simulink model "UPQC_model"  (R2020b)
settings: Solver=FixedStepAuto  StartTime=0.0  StopTime=Tsim  FixedStep=Tsample  MaxStep=Tsample  RelTol=1e-3
values from neighbouring files (symbols this model uses):
  C_parallel_Series = zeros(1,4)    [Netzmodell_Ini_DL.m]    (also in workspace_Ini.mat = [1e-05 1e-05 1e-05 0])
  C_parallel_Shunt = zeros(1,4)    [Netzmodell_Ini_DL.m]    (also in workspace_Ini.mat = [1e-05 1e-05 1e-05 0])
  CC_Ki = 5    [Netzmodell_Ini_DL.m]    (also in workspace_Ini.mat)
  CC_Ki_geg = 5    [Netzmodell_Ini_DL.m]    (also in workspace_Ini.mat)
  CC_Kp = 10    [Netzmodell_Ini_DL.m]    (also in workspace_Ini.mat)
  CC_Kp_geg = 10    [Netzmodell_Ini_DL.m]    (also in workspace_Ini.mat)
  CC_OS =     [workspace_Ini.mat]
  Czk = Szenario.Czk*u    [Netzmodell_Ini_DL.m]    (also in workspace_Ini.mat = 0.003)
  fak_RVC = Szenario.fak_RVC    [Netzmodell_Ini_DL.m]    (also in workspace_Ini.mat = [1 1 1])
  fak_Uns = [1; 1; 1]    [Netzmodell_Ini_DL.m]    (also in workspace_Ini.mat = [1 1 1])
  Flicker_Schaltzeitpunkte_L1 = Schaltzeitpunkte(1,:)    [Netzmodell_Ini_DL.m]    (also in workspace_Ini.mat = 10.5)
  Flicker_Schaltzeitpunkte_L2 = Schaltzeitpunkte(2,:)    [Netzmodell_Ini_DL.m]    (also in workspace_Ini.mat = 10.5)
  Flicker_Schaltzeitpunkte_L3 = Schaltzeitpunkte(3,:)    [Netzmodell_Ini_DL.m]    (also in workspace_Ini.mat = 10.5)
  fs = [f_nom; f_nom; f_nom]    [Netzmodell_Ini_DL.m]    (also in workspace_Ini.mat = [50 50 50])
  fsw = Szenario.fsw*k    [Netzmodell_Ini_DL.m]    (also in workspace_Ini.mat = 20000)
  I_Basis_Ober_L1 = I_Basis_Ober(1)    [Netzmodell_Ini_DL.m]    (also in workspace_Ini.mat = 0)
  I_Basis_Ober_L2 = I_Basis_Ober(2)    [Netzmodell_Ini_DL.m]    (also in workspace_Ini.mat = 0)
  I_Basis_Ober_L3 = I_Basis_Ober(3)    [Netzmodell_Ini_DL.m]    (also in workspace_Ini.mat = 0)
  I_relativ_Ober_L1 = Szenario.I_relativ_Ober_L1    [Netzmodell_Ini_DL.m]    (also in workspace_Ini.mat = [0 100 0 100 100 0 100 100 0 0 0 0 ... (50 elements, 1x50)])
  I_relativ_Ober_L2 = Szenario.I_relativ_Ober_L2    [Netzmodell_Ini_DL.m]    (also in workspace_Ini.mat = [0 100 0 100 100 0 100 100 0 0 0 0 ... (50 elements, 1x50)])
  I_relativ_Ober_L3 = Szenario.I_relativ_Ober_L3    [Netzmodell_Ini_DL.m]    (also in workspace_Ini.mat = [0 100 0 100 100 0 100 100 0 0 0 0 ... (50 elements, 1x50)])
  L_Ausgang_Series = zeros(1,4)    [Netzmodell_Ini_DL.m]    (also in workspace_Ini.mat = [0.00093 0.00093 0.00093 0.00093])
  L_Ausgang_Shunt = zeros(1,4)    [Netzmodell_Ini_DL.m]    (also in workspace_Ini.mat = [0.00093 0.00093 0.00093 0.00093])
  L_Eingang_Series = zeros(1,4)    [Netzmodell_Ini_DL.m]    (also in workspace_Ini.mat = [0.00085 0.00085 0.00085 0.00085])
  L_Eingang_Shunt = zeros(1,4)    [Netzmodell_Ini_DL.m]    (also in workspace_Ini.mat = [0.00085 0.00085 0.00085 0.00085])
  Ls_in = 52.2*u/10    (= 5.22e-06)    [Netzmodell_Ini_DL.m]    (also in workspace_Ini.mat)
  Ltrans = Szenario.Ltrans*m    [Netzmodell_Ini_DL.m]    (also in workspace_Ini.mat = 0.000256)
  OS_off = 6    [Netzmodell_Ini_DL.m]    (also in workspace_Ini.mat)
  OS_on = 1    [Netzmodell_Ini_DL.m]    (also in workspace_Ini.mat)
  Phi_Ober_L1 = Phi_Ober(1)    [Netzmodell_Ini_DL.m]    (also in workspace_Ini.mat = 0)
  Phi_Ober_L2 = Phi_Ober(2)    [Netzmodell_Ini_DL.m]    (also in workspace_Ini.mat = -120)
  Phi_Ober_L3 = Phi_Ober(3)    [Netzmodell_Ini_DL.m]    (also in workspace_Ini.mat = 120)
  Phis = [0; -120; 120]    [Netzmodell_Ini_DL.m]    (also in workspace_Ini.mat = [0 -120 120])
  Pl_Flicker = Pl_Flicker*k    [Netzmodell_Ini_DL.m]    (also in workspace_Ini.mat = [5000 5000 5000])
  Pl_Grund = Szenario.Pl_Grund *k    [Netzmodell_Ini_DL.m]    (also in workspace_Ini.mat = [5 5 5])
  Pl_RVC = Pl_RVC*k    [Netzmodell_Ini_DL.m]    (also in workspace_Ini.mat = [10000 10000 10000])
  Pl_Uns = Pl_Uns*k    [Netzmodell_Ini_DL.m]    (also in workspace_Ini.mat = [25000 10 10])
  Ql_ind_Flicker = Ql_ind_Flicker*k    [Netzmodell_Ini_DL.m]    (also in workspace_Ini.mat = [0 0 0])
  Ql_ind_Grund = Szenario.Ql_ind_Grund*k    [Netzmodell_Ini_DL.m]    (also in workspace_Ini.mat = [0 0 0])
  Ql_ind_RVC = Szenario.Ql_ind_RVC*k    [Netzmodell_Ini_DL.m]    (also in workspace_Ini.mat = [0 0 0])
  Ql_ind_Uns = Ql_ind_Uns*k    [Netzmodell_Ini_DL.m]    (also in workspace_Ini.mat = [0 0 0])
  Ql_kap_Flicker = Ql_kap_Flicker*k    [Netzmodell_Ini_DL.m]    (also in workspace_Ini.mat = [0 0 0])
  Ql_kap_Grund = Szenario.Ql_kap_Grund*k    [Netzmodell_Ini_DL.m]    (also in workspace_Ini.mat = [0 0 0])
  Ql_kap_RVC = Szenario.Ql_kap_RVC*k    [Netzmodell_Ini_DL.m]    (also in workspace_Ini.mat = [0 0 0])
  Ql_kap_Uns = Ql_kap_Uns*k    [Netzmodell_Ini_DL.m]    (also in workspace_Ini.mat = [0 0 0])
  R_Ausgang_Series = zeros(1,4)    [Netzmodell_Ini_DL.m]    (also in workspace_Ini.mat = [0.1 0.1 0.1 0.1])
  R_Ausgang_Shunt = zeros(1,4)    [Netzmodell_Ini_DL.m]    (also in workspace_Ini.mat = [0.1 0.1 0.1 0.1])
  R_Eingang_Series = zeros(1,4)    [Netzmodell_Ini_DL.m]    (also in workspace_Ini.mat = [0.1 0.1 0.1 0.1])
  R_Eingang_Shunt = zeros(1,4)    [Netzmodell_Ini_DL.m]    (also in workspace_Ini.mat = [0.1 0.1 0.1 0.1])
  R_parallel_Series = zeros(1,4)    [Netzmodell_Ini_DL.m]    (also in workspace_Ini.mat = [13 13 13 0])
  R_parallel_Shunt = zeros(1,4)    [Netzmodell_Ini_DL.m]    (also in workspace_Ini.mat = [13 13 13 0])
  R_ZK_Belastung = 20    [Netzmodell_Ini_DL.m]    (also in workspace_Ini.mat)
  Rs_in = 5.2*m/10    (= 0.00052)    [Netzmodell_Ini_DL.m]    (also in workspace_Ini.mat)
  Rtrans = Szenario.Rtrans    [Netzmodell_Ini_DL.m]    (also in workspace_Ini.mat = 0.206)
  RVC_L1_on_off_Zeitpunkte = Szenario.RVC_L1_on_off_Zeitpunkte    [Netzmodell_Ini_DL.m]    (also in workspace_Ini.mat = [10.5 40 10 11 12 13 14 15])
  RVC_L2_on_off_Zeitpunkte = Szenario.RVC_L2_on_off_Zeitpunkte    [Netzmodell_Ini_DL.m]    (also in workspace_Ini.mat = [10.5 40 10 11 12 13 14 15])
  RVC_L3_on_off_Zeitpunkte = Szenario.RVC_L3_on_off_Zeitpunkte    [Netzmodell_Ini_DL.m]    (also in workspace_Ini.mat = [10.5 40 10 11 12 13 14 15])
  RVC_off = 20.5    [Netzmodell_Ini_DL.m]    (also in workspace_Ini.mat)
  RVC_on = 20    [Netzmodell_Ini_DL.m]    (also in workspace_Ini.mat)
  RVC_val = [0.8,0.8,0.8]    [Netzmodell_Ini_DL.m]    (also in workspace_Ini.mat = [0.8 0.8 0.8])
  strans = Szenario.strans    [Netzmodell_Ini_DL.m]    (also in workspace_Ini.mat = 0.25)
  t_breaker_series = tacts    [Netzmodell_Ini_DL.m]    (also in workspace_Ini.mat = 0.5)
  tact = Szenario.tact    [Netzmodell_Ini_DL.m]    (also in workspace_Ini.mat = 0.5)
  tact_OS_Regler = Szenario.tact_OS_Regler    [Netzmodell_Ini_DL.m]    (also in workspace_Ini.mat = 0.5)
  tact_QU = 10    [Netzmodell_Ini_DL.m]    (also in workspace_Ini.mat)
  tacts = Szenario.tacts    [Netzmodell_Ini_DL.m]    (also in workspace_Ini.mat = 0.5)
  Tsample = Szenario.Tsample    [Netzmodell_Ini_DL.m]    (also in workspace_Ini.mat = 5e-06)
  Uns_L1_on_off_Zeitpunkte = Szenario.Uns_L1_on_off_Zeitpunkte    [Netzmodell_Ini_DL.m]    (also in workspace_Ini.mat = [1 6 10 11 12 13 14 15])
  Uns_L2_on_off_Zeitpunkte = Szenario.Uns_L2_on_off_Zeitpunkte    [Netzmodell_Ini_DL.m]    (also in workspace_Ini.mat = [10 30 10 11 12 13 14 15])
  Uns_L3_on_off_Zeitpunkte = Szenario.Uns_L3_on_off_Zeitpunkte    [Netzmodell_Ini_DL.m]    (also in workspace_Ini.mat = [10 30 10 11 12 13 14 15])
  Us = [Us_Amp; Us_Amp; Us_Amp]    [Netzmodell_Ini_DL.m]    (also in workspace_Ini.mat = [326.598632371 326.598632371 326.598632371])
  Us_Amp = sqrt(2)*400/sqrt(3)    [Netzmodell_Ini_DL.m]    (also in workspace_Ini.mat = 326.598632371)
  VC_Ki_gegen = 30    [Netzmodell_Ini_DL.m]    (also in workspace_Ini.mat)
  VC_Ki_gegen_shunt = 15    [Netzmodell_Ini_DL.m]    (also in workspace_Ini.mat)
  VC_Ki_mit = 5    [Netzmodell_Ini_DL.m]    (also in workspace_Ini.mat)
  VC_Kp_gegen = 5    [workspace_Ini.mat]
  VC_Kp_gegen_shunt = 2    [Netzmodell_Ini_DL.m]    (also in workspace_Ini.mat)
  VC_Kp_mit = 10    [Netzmodell_Ini_DL.m]    (also in workspace_Ini.mat)
  VC_ZK_Ki = 5    [Netzmodell_Ini_DL.m]    (also in workspace_Ini.mat)
  VC_ZK_Kp = 0.5    [Netzmodell_Ini_DL.m]    (also in workspace_Ini.mat)
  Vielfache_Ober_L1 = Szenario.Vielfache_Ober_L1    [Netzmodell_Ini_DL.m]    (also in workspace_Ini.mat = [1 2 3 4 5 6 7 8 9 10 11 12 ... (50 elements, 1x50)])
  Vielfache_Ober_L2 = Szenario.Vielfache_Ober_L2    [Netzmodell_Ini_DL.m]    (also in workspace_Ini.mat = [1 2 3 4 5 6 7 8 9 10 11 12 ... (50 elements, 1x50)])
  Vielfache_Ober_L3 = Szenario.Vielfache_Ober_L3    [Netzmodell_Ini_DL.m]    (also in workspace_Ini.mat = [1 2 3 4 5 6 7 8 9 10 11 12 ... (50 elements, 1x50)])
  ZK_Belastung_off = 100    [Netzmodell_Ini_DL.m]    (also in workspace_Ini.mat)
  ZK_Belastung_on = 100    [Netzmodell_Ini_DL.m]    (also in workspace_Ini.mat)
  Zwischenkreisspannung = 700    [Netzmodell_Ini_DL.m]    (also in workspace_Ini.mat)
undefined symbols (not defined in the file or in its folder): LAusgang, RReiheL3
libraries: powerlib x221, powerlib_meascontrol x80, pid_lib x23, eeTransforms x4, eePwmGeneratorTwoLevel x2, dspstat3 x1
(part 3 of 16)

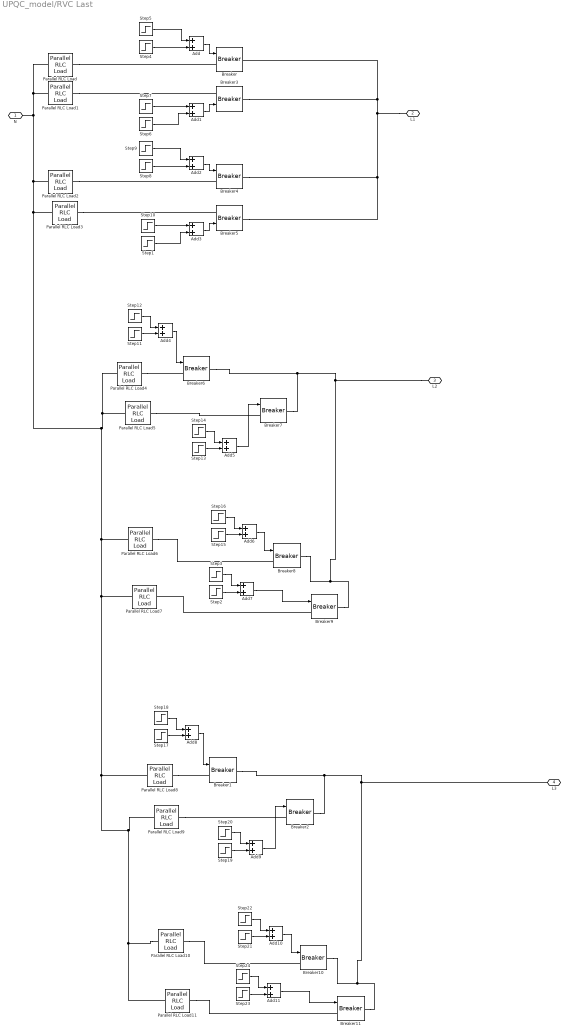
== system UPQC_model/RVC Last ==
  Add{,1..11} (12 alike) : Sum
  Breaker{,1..11} (12 alike) : powerlib/Elements/Breaker  InitialState=0  SwitchingTimes="[1/60  5/60]"  External=on  BreakerResistance=0.01  SnubberResistance=1e6  SnubberCapacitance=inf  Measurements=None  MoreParameters=on  NoBreakLoop=off
  Parallel RLC Load : powerlib/Elements/Parallel RLC Load  LConnTagsString=a  RConnTagsString=__new0  NominalVoltage=230.9  NominalFrequency=50  ActivePower=wirk_L1  InductivePower=blind_ind_L1  CapacitivePower=blind_kap_L1  Setx0=off  InitialVoltage=0  SetiL0=off  InitialCurrent=0  Measurements=None  LoadType=constant Z
      settings: AttributesFormatString=\n  SourceProductBaseCode=PS
  Parallel RLC Load1 : powerlib/Elements/Parallel RLC Load  LConnTagsString=a  RConnTagsString=__new0  NominalVoltage=230.9  NominalFrequency=50  ActivePower=wirk_L1*faktor_L1  InductivePower=blind_ind_L1*faktor_L1  CapacitivePower=blind_kap_L1*faktor_L1  Setx0=off  InitialVoltage=0  SetiL0=off  InitialCurrent=0  Measurements=None  LoadType=constant Z
      settings: AttributesFormatString=\n  SourceProductBaseCode=PS
  Parallel RLC Load10 : powerlib/Elements/Parallel RLC Load  LConnTagsString=a  RConnTagsString=__new0  NominalVoltage=230.9  NominalFrequency=50  ActivePower=wirk_L3*faktor_L3*faktor_L3  InductivePower=blind_ind_L3*faktor_L3*faktor_L3  CapacitivePower=blind_kap_L3*faktor_L3*faktor_L3  Setx0=off  InitialVoltage=0  SetiL0=off  InitialCurrent=0  Measurements=None  LoadType=constant Z
      settings: AttributesFormatString=\n  SourceProductBaseCode=PS
  Parallel RLC Load11 : powerlib/Elements/Parallel RLC Load  LConnTagsString=a  RConnTagsString=__new0  NominalVoltage=230.9  NominalFrequency=50  ActivePower=wirk_L3*faktor_L3*faktor_L3*faktor_L3  InductivePower=blind_ind_L3*faktor_L3*faktor_L3*faktor_L3  CapacitivePower=blind_kap_L3*faktor_L3*faktor_L3*faktor_L3  Setx0=off  InitialVoltage=0  SetiL0=off  InitialCurrent=0  Measurements=None  LoadType=constant Z
      settings: AttributesFormatString=\n  SourceProductBaseCode=PS
  Parallel RLC Load2 : powerlib/Elements/Parallel RLC Load  LConnTagsString=a  RConnTagsString=__new0  NominalVoltage=230.9  NominalFrequency=50  ActivePower=wirk_L1*faktor_L1*faktor_L1  InductivePower=blind_ind_L1*faktor_L1*faktor_L1  CapacitivePower=blind_kap_L1*faktor_L1*faktor_L1  Setx0=off  InitialVoltage=0  SetiL0=off  InitialCurrent=0  Measurements=None  LoadType=constant Z
      settings: AttributesFormatString=\n  SourceProductBaseCode=PS
  Parallel RLC Load3 : powerlib/Elements/Parallel RLC Load  LConnTagsString=a  RConnTagsString=__new0  NominalVoltage=230.9  NominalFrequency=50  ActivePower=wirk_L1*faktor_L1*faktor_L1*faktor_L1  InductivePower=blind_ind_L1*faktor_L1*faktor_L1*faktor_L1  CapacitivePower=blind_kap_L1*faktor_L1*faktor_L1*faktor_L1  Setx0=off  InitialVoltage=0  SetiL0=off  InitialCurrent=0  Measurements=None  LoadType=constant Z
      settings: AttributesFormatString=\n  SourceProductBaseCode=PS
  Parallel RLC Load4 : powerlib/Elements/Parallel RLC Load  LConnTagsString=a  RConnTagsString=__new0  NominalVoltage=230.9  NominalFrequency=50  ActivePower=wirk_L2  InductivePower=blind_ind_L2  CapacitivePower=blind_kap_L2  Setx0=off  InitialVoltage=0  SetiL0=off  InitialCurrent=0  Measurements=None  LoadType=constant Z
      settings: AttributesFormatString=\n  SourceProductBaseCode=PS
  Parallel RLC Load5 : powerlib/Elements/Parallel RLC Load  LConnTagsString=a  RConnTagsString=__new0  NominalVoltage=230.9  NominalFrequency=50  ActivePower=wirk_L2*faktor_L2  InductivePower=blind_ind_L2*faktor_L2  CapacitivePower=blind_kap_L2*faktor_L2  Setx0=off  InitialVoltage=0  SetiL0=off  InitialCurrent=0  Measurements=None  LoadType=constant Z
      settings: AttributesFormatString=\n  SourceProductBaseCode=PS
  Parallel RLC Load6 : powerlib/Elements/Parallel RLC Load  LConnTagsString=a  RConnTagsString=__new0  NominalVoltage=230.9  NominalFrequency=50  ActivePower=wirk_L2*faktor_L2*faktor_L2  InductivePower=blind_ind_L2*faktor_L2*faktor_L2  CapacitivePower=blind_kap_L2*faktor_L2*faktor_L2  Setx0=off  InitialVoltage=0  SetiL0=off  InitialCurrent=0  Measurements=None  LoadType=constant Z
      settings: AttributesFormatString=\n  SourceProductBaseCode=PS
  Parallel RLC Load7 : powerlib/Elements/Parallel RLC Load  LConnTagsString=a  RConnTagsString=__new0  NominalVoltage=230.9  NominalFrequency=50  ActivePower=wirk_L2*faktor_L2*faktor_L2*faktor_L2  InductivePower=blind_ind_L2*faktor_L2*faktor_L2*faktor_L2  CapacitivePower=blind_kap_L2*faktor_L2*faktor_L2*faktor_L2  Setx0=off  InitialVoltage=0  SetiL0=off  InitialCurrent=0  Measurements=None  LoadType=constant Z
      settings: AttributesFormatString=\n  SourceProductBaseCode=PS
  Parallel RLC Load8 : powerlib/Elements/Parallel RLC Load  LConnTagsString=a  RConnTagsString=__new0  NominalVoltage=230.9  NominalFrequency=50  ActivePower=wirk_L3  InductivePower=blind_ind_L3  CapacitivePower=blind_kap_L3  Setx0=off  InitialVoltage=0  SetiL0=off  InitialCurrent=0  Measurements=None  LoadType=constant Z
      settings: AttributesFormatString=\n  SourceProductBaseCode=PS
  Parallel RLC Load9 : powerlib/Elements/Parallel RLC Load  LConnTagsString=a  RConnTagsString=__new0  NominalVoltage=230.9  NominalFrequency=50  ActivePower=wirk_L3*faktor_L3  InductivePower=blind_ind_L3*faktor_L3  CapacitivePower=blind_kap_L3*faktor_L3  Setx0=off  InitialVoltage=0  SetiL0=off  InitialCurrent=0  Measurements=None  LoadType=constant Z
      settings: AttributesFormatString=\n  SourceProductBaseCode=PS
  Step1 : Step  Time=t4_L1  SampleTime=0
  Step10 : Step  Time=t4_L1+(t4_L1_off-t4_L1)  After=-1  SampleTime=0
  Step11 : Step  Time=t1_L2  SampleTime=0
  Step12 : Step  Time=t1_L2+(t1_L2_off-t1_L2)  After=-1  SampleTime=0
  Step13 : Step  Time=t2_L2  SampleTime=0
  Step14 : Step  Time=t2_L2+(t2_L2_off-t2_L2)  After=-1  SampleTime=0
  Step15 : Step  Time=t3_L2  SampleTime=0
  Step16 : Step  Time=t3_L2+(t3_L2_off-t3_L2)  After=-1  SampleTime=0
  Step17 : Step  Time=t1_L3  SampleTime=0
  Step18 : Step  Time=t1_L3+(t1_L3_off-t1_L3)  After=-1  SampleTime=0
  Step19 : Step  Time=t2_L3  SampleTime=0
  Step2 : Step  Time=t4_L2  SampleTime=0
  Step20 : Step  Time=t2_L3+(t2_L3_off-t2_L3)  After=-1  SampleTime=0
  Step21 : Step  Time=t3_L3  SampleTime=0
  Step22 : Step  Time=t3_L3+(t3_L3_off-t3_L3)  After=-1  SampleTime=0
  Step23 : Step  Time=t4_L3  SampleTime=0
  Step24 : Step  Time=t4_L3+(t4_L3_off-t4_L3)  After=-1  SampleTime=0
  Step3 : Step  Time=t4_L2+(t4_L2_off-t4_L2)  After=-1  SampleTime=0
  Step4 : Step  Time=t1_L1  SampleTime=0
  Step5 : Step  Time=t1_L1+(t1_L1_off-t1_L1)  After=-1  SampleTime=0
  Step6 : Step  Time=t2_L1  SampleTime=0
  Step7 : Step  Time=t2_L1+(t2_L1_off-t2_L1)  After=-1  SampleTime=0
  Step8 : Step  Time=t3_L1  SampleTime=0
  Step9 : Step  Time=t3_L1+(t3_L1_off-t3_L1)  After=-1  SampleTime=0
  N : PMIOPort  Side=Left
  L1 : PMIOPort  Port=2  Side=Right
  L2 : PMIOPort  Port=3  Side=Right
  L3 : PMIOPort  Port=4  Side=Right
  wires:
  Step19/1 -> Add9/2
  Step18/1 -> Add8/1
  Step22/1 -> Add10/1
  Step24/1 -> Add11/1
  Step21/1 -> Add10/2
  Add8/1 -> Breaker1/1
  Add11/1 -> Breaker11/1
  Step23/1 -> Add11/2
  Add9/1 -> Breaker2/1
  Step20/1 -> Add9/1
  Step17/1 -> Add8/2
  Add10/1 -> Breaker10/1
  Step11/1 -> Add4/2
  Step14/1 -> Add5/1
  Step13/1 -> Add5/2
  Add6/1 -> Breaker8/1
  Step15/1 -> Add6/2
  Step12/1 -> Add4/1
  Add4/1 -> Breaker6/1
  Add7/1 -> Breaker9/1
  Step16/1 -> Add6/1
  Add5/1 -> Breaker7/1
  Step2/1 -> Add7/2
  Step3/1 -> Add7/1
  Add3/1 -> Breaker5/1
  Step1/1 -> Add3/2
  Step10/1 -> Add3/1
  Add2/1 -> Breaker4/1
  Step8/1 -> Add2/2
  Step9/1 -> Add2/1
  Step7/1 -> Add1/1
  Step6/1 -> Add1/2
  Add1/1 -> Breaker3/1
  Add/1 -> Breaker/1
  Step4/1 -> Add/2
  Step5/1 -> Add/1
  connections:
  Parallel RLC Load10/RConn1 -- Breaker10/LConn1
  Parallel RLC Load9/RConn1 -- Breaker2/LConn1
  Parallel RLC Load11/RConn1 -- Breaker11/LConn1
  Parallel RLC Load8/RConn1 -- Breaker1/LConn1
  Breaker2/RConn1 -- Breaker1/RConn1 -- L3/RConn1 -- Breaker10/RConn1 -- Breaker11/RConn1
  Parallel RLC Load6/RConn1 -- Breaker8/LConn1
  Parallel RLC Load4/RConn1 -- Breaker6/LConn1
  Breaker9/LConn1 -- Parallel RLC Load7/RConn1
  Parallel RLC Load5/RConn1 -- Breaker7/LConn1
  L2/RConn1 -- Breaker7/RConn1 -- Breaker6/RConn1 -- Breaker8/RConn1 -- Breaker9/RConn1
  Parallel RLC Load3/RConn1 -- Breaker5/LConn1
  Parallel RLC Load2/RConn1 -- Breaker4/LConn1
  Parallel RLC Load1/RConn1 -- Breaker3/LConn1
  Parallel RLC Load/RConn1 -- Breaker/LConn1
  L1/RConn1 -- Breaker5/RConn1 -- Breaker4/RConn1 -- Breaker/RConn1 -- Breaker3/RConn1
  Parallel RLC Load10/LConn1 -- Parallel RLC Load11/LConn1 -- Parallel RLC Load8/LConn1 -- Parallel RLC Load7/LConn1 -- N/RConn1 -- Parallel RLC Load/LConn1 -- Parallel RLC Load1/LConn1 -- Parallel RLC Load2/LConn1 -- Parallel RLC Load3/LConn1 -- Parallel RLC Load4/LConn1 -- Parallel RLC Load5/LConn1 -- Parallel RLC Load6/LConn1 -- Parallel RLC Load9/LConn1

== system UPQC_model/Series UPQC ==
  Serienkompensator : Subsystem
  Step : Step  Time=tacts  SampleTime=0
  tag scope: Sollwerte_Series_U=global
  wires:
  [Iabc_E] -> Serienkompensator/3(VSC-Strom)
  [Vabc_C] -> Serienkompensator/4(PCC-Spg)
  Step/1 -> Serienkompensator/1(enable)
  Serienkompensator/1(sp) -> [Sollwerte_Series_U]
  [PLL] -> Serienkompensator/2(PLL)

== system UPQC_model/Series UPQC1 ==
  note: Netzsynchronisation
  Subsystem15 : Subsystem
  tag scope: PLL=global
  wires:
  [Vabc_C] -> Subsystem15/1(In1)
  Subsystem15/1(Out5) -> [PLL]

== system UPQC_model/Shunt UPQC ==
  Shuntkompensator : Subsystem
  Step : Step  Time=tact  SampleTime=0
  tag scope: Sollwerte_Shunt_U=global
  wires:
  Step/1 -> Shuntkompensator/1(enable)
  Shuntkompensator/1(sp) -> [Sollwerte_Shunt_U]
  [PLL] -> Shuntkompensator/2(PLL)
  [Vabc_C] -> Shuntkompensator/4(PCC-Spg)
  [Iabc_D] -> Shuntkompensator/3(VSC-Strom)
  [Iabc_C] -> Shuntkompensator/5(Laststrom)

== system UPQC_model/Sollwertquelle_Series_U ==
  Sollwerte_Uabc : Inport
  Controlled Voltage Source3 : powerlib/Electrical Sources/Controlled Voltage Source  Initialize=on  Source_Type=AC  Amplitude=0  Phase=0  Frequency=0  Measurements=None
  Controlled Voltage Source4 : powerlib/Electrical Sources/Controlled Voltage Source  Initialize=on  Source_Type=AC  Amplitude=0  Phase=0  Frequency=0  Measurements=None
  Controlled Voltage Source5 : powerlib/Electrical Sources/Controlled Voltage Source  Initialize=on  Source_Type=AC  Amplitude=0  Phase=0  Frequency=0  Measurements=None
  Demux : Demux  Outputs=3
  Ground : powerlib/Elements/Ground  LConnTagsString=a
  Series RLC Branch : powerlib/Elements/Series RLC Branch  LConnTagsString=__new0  RConnTagsString=__new0  BranchType=R  Resistance=1000000  Inductance=1e-3  SetiL0=off  InitialCurrent=0  Capacitance=1e-6  Setx0=off  InitialVoltage=0  Measurements=None
  Transport Delay : TransportDelay  DelayTime=0.5/fsw
  Transport Delay1 : TransportDelay  DelayTime=0.5/fsw
  Transport Delay2 : TransportDelay  DelayTime=0.5/fsw
  A : PMIOPort  Side=Right
  B : PMIOPort  Port=2  Side=Right
  C : PMIOPort  Port=3  Side=Right
  wires:
  Sollwerte_Uabc/1 -> Demux/1
  Demux/2 -> Transport Delay1/1
  Demux/1 -> Transport Delay/1
  Transport Delay/1 -> Controlled Voltage Source3/1
  Transport Delay1/1 -> Controlled Voltage Source4/1
  Demux/3 -> Transport Delay2/1
  Transport Delay2/1 -> Controlled Voltage Source5/1
  connections:
  B/RConn1 -- Controlled Voltage Source4/RConn1
  A/RConn1 -- Controlled Voltage Source3/RConn1
  Controlled Voltage Source5/RConn1 -- C/RConn1
  Series RLC Branch/RConn1 -- Ground/LConn1
  Controlled Voltage Source5/LConn1 -- Controlled Voltage Source3/LConn1 -- Controlled Voltage Source4/LConn1 -- Series RLC Branch/LConn1

== system UPQC_model/Sollwertquelle_Shunt_U ==
  Sollwerte_Uabc : Inport
  Controlled Voltage Source3 : powerlib/Electrical Sources/Controlled Voltage Source  Initialize=on  Source_Type=AC  Amplitude=0  Phase=0  Frequency=0  Measurements=None
  Controlled Voltage Source4 : powerlib/Electrical Sources/Controlled Voltage Source  Initialize=on  Source_Type=AC  Amplitude=0  Phase=0  Frequency=0  Measurements=None
  Controlled Voltage Source5 : powerlib/Electrical Sources/Controlled Voltage Source  Initialize=on  Source_Type=AC  Amplitude=0  Phase=0  Frequency=0  Measurements=None
  Demux : Demux  Outputs=3
  Ground : powerlib/Elements/Ground  Commented=on  LConnTagsString=a
  Series RLC Branch : powerlib/Elements/Series RLC Branch  LConnTagsString=__new0  RConnTagsString=__new0  BranchType=R  Resistance=10  Inductance=1e-3  SetiL0=off  InitialCurrent=0  Capacitance=1e-6  Setx0=off  InitialVoltage=0  Measurements=None
  Series RLC Branch1 : powerlib/Elements/Series RLC Branch  LConnTagsString=__new0  RConnTagsString=__new0  BranchType=R  Resistance=10  Inductance=1e-3  SetiL0=off  InitialCurrent=0  Capacitance=1e-6  Setx0=off  InitialVoltage=0  Measurements=None
  Series RLC Branch2 : powerlib/Elements/Series RLC Branch  LConnTagsString=__new0  RConnTagsString=__new0  BranchType=R  Resistance=10  Inductance=1e-3  SetiL0=off  InitialCurrent=0  Capacitance=1e-6  Setx0=off  InitialVoltage=0  Measurements=None
  Transport Delay : TransportDelay  DelayTime=0.5/fsw
  Transport Delay1 : TransportDelay  DelayTime=0.5/fsw
  Transport Delay2 : TransportDelay  DelayTime=0.5/fsw
  A : PMIOPort  Side=Right
  B : PMIOPort  Port=2  Side=Right
  C : PMIOPort  Port=3  Side=Right
  wires:
  Sollwerte_Uabc/1 -> Demux/1
  Demux/2 -> Transport Delay1/1
  Demux/1 -> Transport Delay/1
  Transport Delay/1 -> Controlled Voltage Source3/1
  Transport Delay1/1 -> Controlled Voltage Source4/1
  Demux/3 -> Transport Delay2/1
  Transport Delay2/1 -> Controlled Voltage Source5/1
  connections:
  Controlled Voltage Source5/RConn1 -- Series RLC Branch2/RConn1
  Controlled Voltage Source4/RConn1 -- Series RLC Branch1/RConn1
  Controlled Voltage Source3/RConn1 -- Series RLC Branch/RConn1
  Series RLC Branch/LConn1 -- A/RConn1
  Series RLC Branch2/LConn1 -- C/RConn1
  Series RLC Branch1/LConn1 -- B/RConn1
  Controlled Voltage Source5/LConn1 -- Ground/LConn1 -- Controlled Voltage Source4/LConn1 -- Controlled Voltage Source3/LConn1

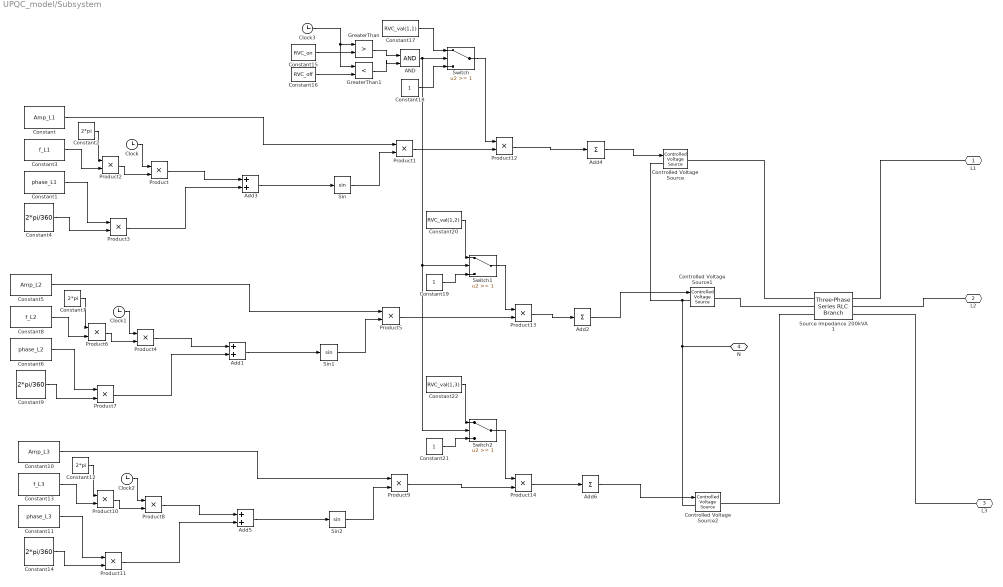
== system UPQC_model/Subsystem ==
  AND : Logic  IconShape=distinctive  AllPortsSameDT=off  OutDataTypeStr=boolean
  Add1 : Sum
  Add2 : Sum  Inputs=+
  Add3 : Sum
  Add4 : Sum  Inputs=+
  Add5 : Sum
  Add6 : Sum  Inputs=+
  Clock{,1..3} (4 alike) : Clock
  Constant : Constant  Value=Amp_L1
  Constant1 : Constant  Value=phase_L1
  Constant10 : Constant  Value=Amp_L3
  Constant11 : Constant  Value=phase_L3
  Constant12 : Constant  Value=2*pi
  Constant13 : Constant  Value=f_L3
  Constant14 : Constant  Value=2*pi/360
  Constant15 : Constant  Value=RVC_on
  Constant16 : Constant  Value=RVC_off
  Constant17 : Constant  Value=RVC_val(1,1)
  Constant18 : Constant
  Constant19 : Constant
  Constant2 : Constant  Value=2*pi
  Constant20 : Constant  Value=RVC_val(1,2)
  Constant21 : Constant
  Constant22 : Constant  Value=RVC_val(1,3)
  Constant3 : Constant  Value=f_L1
  Constant4 : Constant  Value=2*pi/360
  Constant5 : Constant  Value=Amp_L2
  Constant6 : Constant  Value=phase_L2
  Constant7 : Constant  Value=2*pi
  Constant8 : Constant  Value=f_L2
  Constant9 : Constant  Value=2*pi/360
  Controlled Voltage Source : powerlib/Electrical Sources/Controlled Voltage Source  Initialize=on  Source_Type=AC  Amplitude=0  Phase=0  Frequency=0  Measurements=None
  Controlled Voltage Source1 : powerlib/Electrical Sources/Controlled Voltage Source  Initialize=on  Source_Type=AC  Amplitude=0  Phase=0  Frequency=0  Measurements=None
  Controlled Voltage Source2 : powerlib/Electrical Sources/Controlled Voltage Source  Initialize=on  Source_Type=AC  Amplitude=0  Phase=0  Frequency=0  Measurements=None
  GreaterThan : RelationalOperator  Operator=>  OutDataTypeStr=boolean  RndMeth=Simplest
  GreaterThan1 : RelationalOperator  Operator=<  OutDataTypeStr=boolean  RndMeth=Simplest
  Product{,1..14} (15 alike) : Product
  Sin : Trigonometry
  Sin1 : Trigonometry
  Sin2 : Trigonometry
  Source impedance 200kVA 1 : powerlib/Elements/Three-Phase Series RLC Branch  LConnTagsString=A|B|C  RConnTagsString=A|B|C  BranchType=RL  Resistance=R/10  Inductance=L/10  Capacitance=[]  Measurements=None
  Switch : Switch  Threshold=1
  Switch1 : Switch  Threshold=1
  Switch2 : Switch  Threshold=1
  L1 : PMIOPort  Side=Right
  L2 : PMIOPort  Port=2  Side=Right
  L3 : PMIOPort  Port=3  Side=Right
  N : PMIOPort  Port=4  Side=Right
  wires:
  Constant13/1 -> Product10/2
  Add5/1 -> Sin2/1
  Product8/1 -> Add5/1
  Constant12/1 -> Product10/1
  Product10/1 -> Product8/2
  Sin2/1 -> Product9/2
  Constant11/1 -> Product11/1
  Constant10/1 -> Product9/1
  Clock2/1 -> Product8/1
  Product11/1 -> Add5/2
  Constant14/1 -> Product11/2
  Constant8/1 -> Product6/2
  Add1/1 -> Sin1/1
  Product4/1 -> Add1/1
  Constant7/1 -> Product6/1
  Product6/1 -> Product4/2
  Sin1/1 -> Product5/2
  Constant6/1 -> Product7/1
  Constant5/1 -> Product5/1
  Clock1/1 -> Product4/1
  Product7/1 -> Add1/2
  Constant9/1 -> Product7/2
  Product3/1 -> Add3/2
  Constant4/1 -> Product3/2
  Constant1/1 -> Product3/1
  Product2/1 -> Product/2
  Constant3/1 -> Product2/2
  Constant2/1 -> Product2/1
  Sin/1 -> Product1/2
  Add4/1 -> Controlled Voltage Source/1
  Add2/1 -> Controlled Voltage Source1/1
  Constant/1 -> Product1/1
  Add6/1 -> Controlled Voltage Source2/1
  Product/1 -> Add3/1
  Add3/1 -> Sin/1
  Clock/1 -> Product/1
  Product1/1 -> Product12/2
  Product12/1 -> Add4/1
  Clock3/1 -> GreaterThan1/1, GreaterThan/1
  Constant16/1 -> GreaterThan1/2
  Constant15/1 -> GreaterThan/2
  GreaterThan/1 -> AND/1
  GreaterThan1/1 -> AND/2
  Constant17/1 -> Switch/1
  Constant18/1 -> Switch/3
  Switch/1 -> Product12/1
  Product13/1 -> Add2/1
  Product5/1 -> Product13/2
  Product14/1 -> Add6/1
  Product9/1 -> Product14/2
  Constant19/1 -> Switch1/3
  Constant20/1 -> Switch1/1
  Switch1/1 -> Product13/1
  AND/1 -> Switch/2, Switch2/2, Switch1/2
  Constant21/1 -> Switch2/3
  Constant22/1 -> Switch2/1
  Switch2/1 -> Product14/1
  connections:
  L3/RConn1 -- Source impedance 200kVA 1/RConn3
  L2/RConn1 -- Source impedance 200kVA 1/RConn2
  L1/RConn1 -- Source impedance 200kVA 1/RConn1
  Source impedance 200kVA 1/LConn3 -- Controlled Voltage Source2/RConn1
  Source impedance 200kVA 1/LConn2 -- Controlled Voltage Source1/RConn1
  Source impedance 200kVA 1/LConn1 -- Controlled Voltage Source/RConn1
  N/RConn1 -- Controlled Voltage Source2/LConn1 -- Controlled Voltage Source/LConn1 -- Controlled Voltage Source1/LConn1

== system UPQC_model/Transformator mit Messung ==
  note: 400
  note: 41.83
  Current Measurement1 : powerlib/Measurements/Current Measurement  PhasorSimulation=off  OutputType=Complex  PSBequivalent=0
  Current Measurement2 : powerlib/Measurements/Current Measurement  PhasorSimulation=off  OutputType=Complex  PSBequivalent=0
  Current Measurement7 : powerlib/Measurements/Current Measurement  PhasorSimulation=off  OutputType=Complex  PSBequivalent=0
  Linear Transformer3 : powerlib/Elements/Linear Transformer  UNITS=SI  NominalPower=[11533 50]  winding1=[400 0.0 0]  winding2=[55.64 0.0 0]  ThreeWindings=off  winding3=[3.15e+05 13171 1677]  RmLm=[3691.9 0.104]  Measurements=None  DataType=on
  Linear Transformer6 : powerlib/Elements/Linear Transformer  UNITS=SI  NominalPower=[11533 50]  winding1=[400 0 0]  winding2=[55.64 0 0]  ThreeWindings=off  winding3=[3.15e+05 13171 1677]  RmLm=[3691.9 0.104]  Measurements=None  DataType=on
  Linear Transformer7 : powerlib/Elements/Linear Transformer  UNITS=SI  NominalPower=[11533 50]  winding1=[400 0 0]  winding2=[55.64 0 0]  ThreeWindings=off  winding3=[3.15e+05 13171 1677]  RmLm=[3691.9 0.104]  Measurements=None  DataType=on
  Mux : Mux  Inputs=3
  Mux1 : Mux  Inputs=3
  Voltage Measurement1 : powerlib/Measurements/Voltage Measurement  PhasorSimulation=off  OutputType=Complex  PSBequivalent=0
  Voltage Measurement2 : powerlib/Measurements/Voltage Measurement  PhasorSimulation=off  OutputType=Complex  PSBequivalent=0
  Voltage Measurement3 : powerlib/Measurements/Voltage Measurement  PhasorSimulation=off  OutputType=Complex  PSBequivalent=0
  A : PMIOPort  Side=Left
  B : PMIOPort  Port=2  Side=Left
  C : PMIOPort  Port=3  Side=Left
  c2 : PMIOPort  Port=4  Side=Right
  c1 : PMIOPort  Port=5  Side=Right
  b2 : PMIOPort  Port=6  Side=Right
  b1 : PMIOPort  Port=7  Side=Right
  a2 : PMIOPort  Port=8  Side=Right
  a1 : PMIOPort  Port=9  Side=Right
  I_W1_W2_W3 : Outport
  U_W1_W2_W3 : Outport  Port=2
  wires:
  Mux/1 -> U_W1_W2_W3/1
  Mux1/1 -> I_W1_W2_W3/1
  Current Measurement2/1 -> Mux1/1
  Current Measurement7/1 -> Mux1/2
  Current Measurement1/1 -> Mux1/3
  Voltage Measurement3/1 -> Mux/1
  Voltage Measurement2/1 -> Mux/2
  Voltage Measurement1/1 -> Mux/3
  connections:
  Voltage Measurement2/LConn1 -- Linear Transformer3/LConn1 -- Current Measurement7/LConn1
  Voltage Measurement3/LConn2 -- B/RConn1 -- Current Measurement7/RConn1 -- Linear Transformer7/LConn2
  Voltage Measurement1/LConn1 -- Linear Transformer6/LConn1 -- Current Measurement1/LConn1
  Voltage Measurement3/LConn1 -- Linear Transformer7/LConn1 -- Current Measurement2/LConn1
  Voltage Measurement1/LConn2 -- Linear Transformer6/LConn2 -- Current Measurement2/RConn1 -- A/RConn1
  Voltage Measurement2/LConn2 -- Linear Transformer3/LConn2 -- C/RConn1 -- Current Measurement1/RConn1
  Linear Transformer6/RConn1 -- c1/RConn1
  Linear Transformer6/RConn2 -- c2/RConn1
  Linear Transformer3/RConn1 -- b1/RConn1
  Linear Transformer3/RConn2 -- b2/RConn1
  a1/RConn1 -- Linear Transformer7/RConn1
  Linear Transformer7/RConn2 -- a2/RConn1

== system UPQC_model/Unsymmetrie Last ==
  Add{,1..11} (12 alike) : Sum
  Breaker{,1..11} (12 alike) : powerlib/Elements/Breaker  InitialState=0  SwitchingTimes="[1/60  5/60]"  External=on  BreakerResistance=0.01  SnubberResistance=1e6  SnubberCapacitance=inf  Measurements=None  MoreParameters=on  NoBreakLoop=off
  Parallel RLC Load : powerlib/Elements/Parallel RLC Load  LConnTagsString=a  RConnTagsString=__new0  NominalVoltage=230.9  NominalFrequency=50  ActivePower=wirk_L1  InductivePower=blind_ind_L1  CapacitivePower=blind_kap_L1  Setx0=off  InitialVoltage=0  SetiL0=off  InitialCurrent=0  Measurements=None  LoadType=constant Z
      settings: AttributesFormatString=\n  SourceProductBaseCode=PS
  Parallel RLC Load1 : powerlib/Elements/Parallel RLC Load  LConnTagsString=a  RConnTagsString=__new0  NominalVoltage=230.9  NominalFrequency=50  ActivePower=wirk_L1*faktor_L1  InductivePower=blind_ind_L1*faktor_L1  CapacitivePower=blind_kap_L1*faktor_L1  Setx0=off  InitialVoltage=0  SetiL0=off  InitialCurrent=0  Measurements=None  LoadType=constant Z
      settings: AttributesFormatString=\n  SourceProductBaseCode=PS
  Parallel RLC Load10 : powerlib/Elements/Parallel RLC Load  LConnTagsString=a  RConnTagsString=__new0  NominalVoltage=230.9  NominalFrequency=50  ActivePower=wirk_L3*faktor_L3*faktor_L3  InductivePower=blind_ind_L3*faktor_L3*faktor_L3  CapacitivePower=blind_kap_L3*faktor_L3*faktor_L3  Setx0=off  InitialVoltage=0  SetiL0=off  InitialCurrent=0  Measurements=None  LoadType=constant Z
      settings: AttributesFormatString=\n  SourceProductBaseCode=PS
  Parallel RLC Load11 : powerlib/Elements/Parallel RLC Load  LConnTagsString=a  RConnTagsString=__new0  NominalVoltage=230.9  NominalFrequency=50  ActivePower=wirk_L3*faktor_L3*faktor_L3*faktor_L3  InductivePower=blind_ind_L3*faktor_L3*faktor_L3*faktor_L3  CapacitivePower=blind_kap_L3*faktor_L3*faktor_L3*faktor_L3  Setx0=off  InitialVoltage=0  SetiL0=off  InitialCurrent=0  Measurements=None  LoadType=constant Z
      settings: AttributesFormatString=\n  SourceProductBaseCode=PS
  Parallel RLC Load2 : powerlib/Elements/Parallel RLC Load  LConnTagsString=a  RConnTagsString=__new0  NominalVoltage=230.9  NominalFrequency=50  ActivePower=wirk_L1*faktor_L1*faktor_L1  InductivePower=blind_ind_L1*faktor_L1*faktor_L1  CapacitivePower=blind_kap_L1*faktor_L1*faktor_L1  Setx0=off  InitialVoltage=0  SetiL0=off  InitialCurrent=0  Measurements=None  LoadType=constant Z
      settings: AttributesFormatString=\n  SourceProductBaseCode=PS
  Parallel RLC Load3 : powerlib/Elements/Parallel RLC Load  LConnTagsString=a  RConnTagsString=__new0  NominalVoltage=230.9  NominalFrequency=50  ActivePower=wirk_L1*faktor_L1*faktor_L1*faktor_L1  InductivePower=blind_ind_L1*faktor_L1*faktor_L1*faktor_L1  CapacitivePower=blind_kap_L1*faktor_L1*faktor_L1*faktor_L1  Setx0=off  InitialVoltage=0  SetiL0=off  InitialCurrent=0  Measurements=None  LoadType=constant Z
      settings: AttributesFormatString=\n  SourceProductBaseCode=PS
  Parallel RLC Load4 : powerlib/Elements/Parallel RLC Load  LConnTagsString=a  RConnTagsString=__new0  NominalVoltage=230.9  NominalFrequency=50  ActivePower=wirk_L2  InductivePower=blind_ind_L2  CapacitivePower=blind_kap_L2  Setx0=off  InitialVoltage=0  SetiL0=off  InitialCurrent=0  Measurements=None  LoadType=constant Z
      settings: AttributesFormatString=\n  SourceProductBaseCode=PS
  Parallel RLC Load5 : powerlib/Elements/Parallel RLC Load  LConnTagsString=a  RConnTagsString=__new0  NominalVoltage=230.9  NominalFrequency=50  ActivePower=wirk_L2*faktor_L2  InductivePower=blind_ind_L2*faktor_L2  CapacitivePower=blind_kap_L2*faktor_L2  Setx0=off  InitialVoltage=0  SetiL0=off  InitialCurrent=0  Measurements=None  LoadType=constant Z
      settings: AttributesFormatString=\n  SourceProductBaseCode=PS
  Parallel RLC Load6 : powerlib/Elements/Parallel RLC Load  LConnTagsString=a  RConnTagsString=__new0  NominalVoltage=230.9  NominalFrequency=50  ActivePower=wirk_L2*faktor_L2*faktor_L2  InductivePower=blind_ind_L2*faktor_L2*faktor_L2  CapacitivePower=blind_kap_L2*faktor_L2*faktor_L2  Setx0=off  InitialVoltage=0  SetiL0=off  InitialCurrent=0  Measurements=None  LoadType=constant Z
      settings: AttributesFormatString=\n  SourceProductBaseCode=PS
  Parallel RLC Load7 : powerlib/Elements/Parallel RLC Load  LConnTagsString=a  RConnTagsString=__new0  NominalVoltage=230.9  NominalFrequency=50  ActivePower=wirk_L2*faktor_L2*faktor_L2*faktor_L2  InductivePower=blind_ind_L2*faktor_L2*faktor_L2*faktor_L2  CapacitivePower=blind_kap_L2*faktor_L2*faktor_L2*faktor_L2  Setx0=off  InitialVoltage=0  SetiL0=off  InitialCurrent=0  Measurements=None  LoadType=constant Z
      settings: AttributesFormatString=\n  SourceProductBaseCode=PS
  Parallel RLC Load8 : powerlib/Elements/Parallel RLC Load  LConnTagsString=a  RConnTagsString=__new0  NominalVoltage=230.9  NominalFrequency=50  ActivePower=wirk_L3  InductivePower=blind_ind_L3  CapacitivePower=blind_kap_L3  Setx0=off  InitialVoltage=0  SetiL0=off  InitialCurrent=0  Measurements=None  LoadType=constant Z
      settings: AttributesFormatString=\n  SourceProductBaseCode=PS
  Parallel RLC Load9 : powerlib/Elements/Parallel RLC Load  LConnTagsString=a  RConnTagsString=__new0  NominalVoltage=230.9  NominalFrequency=50  ActivePower=wirk_L3*faktor_L3  InductivePower=blind_ind_L3*faktor_L3  CapacitivePower=blind_kap_L3*faktor_L3  Setx0=off  InitialVoltage=0  SetiL0=off  InitialCurrent=0  Measurements=None  LoadType=constant Z
      settings: AttributesFormatString=\n  SourceProductBaseCode=PS
  Step1 : Step  Time=t4_L1  SampleTime=0
  Step10 : Step  Time=t4_L1+(t4_L1_off-t4_L1)  After=-1  SampleTime=0
  Step11 : Step  Time=t1_L2  SampleTime=0
  Step12 : Step  Time=t1_L2+(t1_L2_off-t1_L2)  After=-1  SampleTime=0
  Step13 : Step  Time=t2_L2  SampleTime=0
  Step14 : Step  Time=t2_L2+(t2_L2_off-t2_L2)  After=-1  SampleTime=0
  Step15 : Step  Time=t3_L2  SampleTime=0
  Step16 : Step  Time=t3_L2+(t3_L2_off-t3_L2)  After=-1  SampleTime=0
  Step17 : Step  Time=t1_L3  SampleTime=0
  Step18 : Step  Time=t1_L3+(t1_L3_off-t1_L3)  After=-1  SampleTime=0
  Step19 : Step  Time=t2_L3  SampleTime=0
  Step2 : Step  Time=t4_L2  SampleTime=0
  Step20 : Step  Time=t2_L3+(t2_L3_off-t2_L3)  After=-1  SampleTime=0
  Step21 : Step  Time=t3_L3  SampleTime=0
  Step22 : Step  Time=t3_L3+(t3_L3_off-t3_L3)  After=-1  SampleTime=0
  Step23 : Step  Time=t4_L3  SampleTime=0
  Step24 : Step  Time=t4_L3+(t4_L3_off-t4_L3)  After=-1  SampleTime=0
  Step3 : Step  Time=t4_L2+(t4_L2_off-t4_L2)  After=-1  SampleTime=0
  Step4 : Step  Time=t1_L1  SampleTime=0
  Step5 : Step  Time=t1_L1+(t1_L1_off-t1_L1)  After=-1  SampleTime=0
  Step6 : Step  Time=t2_L1  SampleTime=0
  Step7 : Step  Time=t2_L1+(t2_L1_off-t2_L1)  After=-1  SampleTime=0
  Step8 : Step  Time=t3_L1  SampleTime=0
  Step9 : Step  Time=t3_L1+(t3_L1_off-t3_L1)  After=-1  SampleTime=0
  N : PMIOPort  Side=Left
  L1 : PMIOPort  Port=2  Side=Right
  L2 : PMIOPort  Port=3  Side=Right
  L3 : PMIOPort  Port=4  Side=Right
  wires:
  Step19/1 -> Add9/2
  Step18/1 -> Add8/1
  Step22/1 -> Add10/1
  Step24/1 -> Add11/1
  Step21/1 -> Add10/2
  Add8/1 -> Breaker1/1
  Add11/1 -> Breaker11/1
  Step23/1 -> Add11/2
  Add9/1 -> Breaker2/1
  Step20/1 -> Add9/1
  Step17/1 -> Add8/2
  Add10/1 -> Breaker10/1
  Step11/1 -> Add4/2
  Step14/1 -> Add5/1
  Step13/1 -> Add5/2
  Add6/1 -> Breaker8/1
  Step15/1 -> Add6/2
  Step12/1 -> Add4/1
  Add4/1 -> Breaker6/1
  Add7/1 -> Breaker9/1
  Step16/1 -> Add6/1
  Add5/1 -> Breaker7/1
  Step2/1 -> Add7/2
  Step3/1 -> Add7/1
  Add3/1 -> Breaker5/1
  Step1/1 -> Add3/2
  Step10/1 -> Add3/1
  Add2/1 -> Breaker4/1
  Step8/1 -> Add2/2
  Step9/1 -> Add2/1
  Step7/1 -> Add1/1
  Step6/1 -> Add1/2
  Add1/1 -> Breaker3/1
  Add/1 -> Breaker/1
  Step4/1 -> Add/2
  Step5/1 -> Add/1
  connections:
  Parallel RLC Load10/RConn1 -- Breaker10/LConn1
  Parallel RLC Load9/RConn1 -- Breaker2/LConn1
  Parallel RLC Load11/RConn1 -- Breaker11/LConn1
  Parallel RLC Load8/RConn1 -- Breaker1/LConn1
  Breaker2/RConn1 -- Breaker1/RConn1 -- L3/RConn1 -- Breaker10/RConn1 -- Breaker11/RConn1
  Parallel RLC Load6/RConn1 -- Breaker8/LConn1
  Parallel RLC Load4/RConn1 -- Breaker6/LConn1
  Breaker9/LConn1 -- Parallel RLC Load7/RConn1
  Parallel RLC Load5/RConn1 -- Breaker7/LConn1
  L2/RConn1 -- Breaker7/RConn1 -- Breaker6/RConn1 -- Breaker8/RConn1 -- Breaker9/RConn1
  Parallel RLC Load3/RConn1 -- Breaker5/LConn1
  Parallel RLC Load2/RConn1 -- Breaker4/LConn1
  Parallel RLC Load1/RConn1 -- Breaker3/LConn1
  Parallel RLC Load/RConn1 -- Breaker/LConn1
  L1/RConn1 -- Breaker5/RConn1 -- Breaker4/RConn1 -- Breaker/RConn1 -- Breaker3/RConn1
  Parallel RLC Load10/LConn1 -- Parallel RLC Load11/LConn1 -- Parallel RLC Load8/LConn1 -- Parallel RLC Load7/LConn1 -- N/RConn1 -- Parallel RLC Load/LConn1 -- Parallel RLC Load1/LConn1 -- Parallel RLC Load2/LConn1 -- Parallel RLC Load3/LConn1 -- Parallel RLC Load4/LConn1 -- Parallel RLC Load5/LConn1 -- Parallel RLC Load6/LConn1 -- Parallel RLC Load9/LConn1

== system UPQC_model/VSC_Series_U ==
  Sollwerte_Uabc : Inport
  Bus Selector : BusSelector  Commented=on  OutputSignals=U DC Zwischenkreis1
  Constant : Constant  Value=370
  Demux : Demux  Commented=on  Outputs=3
  From : From  Commented=on  GotoTag=Messung_Zwischenkreis  TagVisibility=global
  Gain : Gain  Commented=on  Gain=vdc/2
  Gain1 : Gain  Commented=on  Gain=vdc/2
  Gain2 : Gain  Commented=on  Gain=vdc/2
  GreaterThan1 : RelationalOperator  Commented=on  Operator=>  OutDataTypeStr=boolean  RndMeth=Simplest
  GreaterThan2 : RelationalOperator  Commented=on  Operator=>  OutDataTypeStr=boolean  RndMeth=Simplest
  GreaterThan3 : RelationalOperator  Commented=on  Operator=>  OutDataTypeStr=boolean  RndMeth=Simplest
  Mux : Mux  Commented=on  Inputs=6
  NOT1 : Logic  Commented=on  Operator=NOT  IconShape=distinctive  AllPortsSameDT=off  OutDataTypeStr=boolean
  NOT2 : Logic  Commented=on  Operator=NOT  IconShape=distinctive  AllPortsSameDT=off  OutDataTypeStr=boolean
  NOT3 : Logic  Commented=on  Operator=NOT  IconShape=distinctive  AllPortsSameDT=off  OutDataTypeStr=boolean
  PWM generator : eePwmGeneratorTwoLevel/PWM Generator (Three-phase, Two-level)  PWMMode=Continuous PWM (CPWM)  CPWMMode=SPWM: sinusoidal PWM  DPWMMode=60 DPWM (+30 degree shift): +30 degree shift from 60 DPWM  fsw=fsw  Ts=Tsample
      settings: SourceProductBaseCode=PS
  Product : Product  Commented=on
  Step : Step  Commented=on  Time=tacts  SampleTime=0
  Subsystem4 : Subsystem
  Terminator : Terminator  Commented=on
  Terminator1 : Terminator  Commented=on
  Terminator2 : Terminator
  Triangle Generator : powerlib_meascontrol/Pulse & Signal Generators/Triangle Generator  Commented=on  Freq=WR_takt/2  Phase=210  Ts=Tsample
  Triangle Generator1 : powerlib_meascontrol/Pulse & Signal Generators/Triangle Generator  Commented=on  Freq=WR_takt/2  Phase=-30  Ts=Tsample
  Triangle Generator2 : powerlib_meascontrol/Pulse & Signal Generators/Triangle Generator  Commented=on  Freq=WR_takt/2  Phase=90  Ts=Tsample
  Universal Bridge : powerlib/Power Electronics/Universal Bridge  Arms=3  SnubberResistance=1e5  SnubberCapacitance=inf  Device=IGBT / Diodes  Ron=0.7e-3  Lon=0  ForwardVoltages="[  0  0  ]"  ForwardVoltage=0  GTOparameters=[ 10e-6 , 20e-6 ]  IGBTparameters=[ 1e-6 , 2e-6 ]  Measurements=None  Measurements_2=None  converterType=Rectifier
  VSC_Series_U_Dreieckssignale_Scope : Scope  NumInputPorts=2
  DC+ : PMIOPort  Side=Left
  DC- : PMIOPort  Port=2  Side=Left
  A : PMIOPort  Port=3  Side=Right
  B : PMIOPort  Port=4  Side=Right
  C : PMIOPort  Port=5  Side=Right
  Gatesignale_(6) : Outport
  wires:
  NOT2/1 -> Mux/1
  Gain1/1 -> GreaterThan3/1
  Gain2/1 -> GreaterThan1/1
  Gain/1 -> VSC_Series_U_Dreieckssignale_Scope/2, GreaterThan2/1
  Triangle Generator1/1 -> Gain/1
  Mux/1 -> Product/2
  NOT3/1 -> Mux/5
  NOT1/1 -> Mux/3
  GreaterThan3/1 -> NOT3/1, Mux/6
  GreaterThan1/1 -> NOT1/1, Mux/4
  GreaterThan2/1 -> Mux/2, NOT2/1
  Demux/3 -> GreaterThan3/2
  Demux/2 -> GreaterThan1/2
  Demux/1 -> VSC_Series_U_Dreieckssignale_Scope/1, GreaterThan2/2
  Triangle Generator/1 -> Gain1/1
  Triangle Generator2/1 -> Gain2/1
  Sollwerte_Uabc/1 -> PWM generator/1, Demux/1
  Step/1 -> Product/1
  PWM generator/1 -> Subsystem4/1(dVdc)
  From/1 -> Bus Selector/1
  Constant/1 -> PWM generator/2
  Bus Selector/1 -> Terminator/1  "<U DC Zwischenkreis1>"
  Subsystem4/1(Gatesignale_(6)) -> Gatesignale_(6)/1, Universal Bridge/1
  Product/1 -> Terminator1/1
  PWM generator/2 -> Terminator2/1
  connections:
  DC-/RConn1 -- Universal Bridge/RConn2
  A/RConn1 -- Universal Bridge/LConn1
  C/RConn1 -- Universal Bridge/LConn3
  DC+/RConn1 -- Universal Bridge/RConn1
  B/RConn1 -- Universal Bridge/LConn2

== system UPQC_model/VSC_Shunt_U ==
  Sollwerte_Uabc : Inport
  Constant1 : Constant  Value=370
  Demux : Demux  Commented=on  Outputs=3
  Gain : Gain  Commented=on  Gain=vdc/2
  Gain1 : Gain  Commented=on  Gain=vdc/2
  Gain2 : Gain  Commented=on  Gain=vdc/2
  GreaterThan1 : RelationalOperator  Commented=on  Operator=>  OutDataTypeStr=boolean  RndMeth=Simplest
  GreaterThan2 : RelationalOperator  Commented=on  Operator=>  OutDataTypeStr=boolean  RndMeth=Simplest
  GreaterThan3 : RelationalOperator  Commented=on  Operator=>  OutDataTypeStr=boolean  RndMeth=Simplest
  Mux : Mux  Commented=on  Inputs=6
  NOT1 : Logic  Commented=on  Operator=NOT  IconShape=distinctive  AllPortsSameDT=off  OutDataTypeStr=boolean
  NOT2 : Logic  Commented=on  Operator=NOT  IconShape=distinctive  AllPortsSameDT=off  OutDataTypeStr=boolean
  NOT3 : Logic  Commented=on  Operator=NOT  IconShape=distinctive  AllPortsSameDT=off  OutDataTypeStr=boolean
  PWM generator : eePwmGeneratorTwoLevel/PWM Generator (Three-phase, Two-level)  PWMMode=Continuous PWM (CPWM)  CPWMMode=SPWM: sinusoidal PWM  DPWMMode=60 DPWM (+30 degree shift): +30 degree shift from 60 DPWM  fsw=fsw  Ts=Tsample
      settings: SourceProductBaseCode=PS
  Subsystem4 : Subsystem
  Terminator : Terminator
  Terminator1 : Terminator  Commented=on
  Triangle Generator : powerlib_meascontrol/Pulse & Signal Generators/Triangle Generator  Commented=on  Freq=WR_takt/2  Phase=210  Ts=Tsample
  Triangle Generator1 : powerlib_meascontrol/Pulse & Signal Generators/Triangle Generator  Commented=on  Freq=WR_takt/2  Phase=-30  Ts=Tsample
  Triangle Generator2 : powerlib_meascontrol/Pulse & Signal Generators/Triangle Generator  Commented=on  Freq=WR_takt/2  Phase=90  Ts=Tsample
  Universal Bridge : powerlib/Power Electronics/Universal Bridge  Arms=3  SnubberResistance=1e5  SnubberCapacitance=inf  Device=IGBT / Diodes  Ron=0.7e-3  Lon=0  ForwardVoltages="[  0  0  ]"  ForwardVoltage=0  GTOparameters=[ 10e-6 , 20e-6 ]  IGBTparameters=[ 1e-6 , 2e-6 ]  Measurements=None  Measurements_2=None  converterType=Rectifier
  DC+ : PMIOPort  Side=Left
  DC- : PMIOPort  Port=2  Side=Left
  A : PMIOPort  Port=3  Side=Right
  B : PMIOPort  Port=4  Side=Right
  C : PMIOPort  Port=5  Side=Right
  Gatesignale_(6) : Outport
  wires:
  Mux/1 -> Terminator1/1
  PWM generator/2 -> Terminator/1
  Subsystem4/1(Gatesignale_(6)) -> Gatesignale_(6)/1, Universal Bridge/1
  PWM generator/1 -> Subsystem4/1(dVdc)
  Constant1/1 -> PWM generator/2
  NOT2/1 -> Mux/1
  Gain1/1 -> GreaterThan3/1
  Gain2/1 -> GreaterThan1/1
  Gain/1 -> GreaterThan2/1
  Triangle Generator1/1 -> Gain/1
  NOT3/1 -> Mux/5
  NOT1/1 -> Mux/3
  GreaterThan3/1 -> NOT3/1, Mux/6
  GreaterThan1/1 -> NOT1/1, Mux/4
  GreaterThan2/1 -> Mux/2, NOT2/1
  Demux/3 -> GreaterThan3/2
  Demux/2 -> GreaterThan1/2
  Demux/1 -> GreaterThan2/2
  Triangle Generator/1 -> Gain1/1
  Triangle Generator2/1 -> Gain2/1
  Sollwerte_Uabc/1 -> Demux/1, PWM generator/1
  connections:
  DC-/RConn1 -- Universal Bridge/RConn2
  A/RConn1 -- Universal Bridge/LConn1
  C/RConn1 -- Universal Bridge/LConn3
  DC+/RConn1 -- Universal Bridge/RConn1
  B/RConn1 -- Universal Bridge/LConn2

== system UPQC_model/Zwischenkreis_Series ==
  C Zwischenkreis : powerlib/Elements/Series RLC Branch  LConnTagsString=__new0  RConnTagsString=__new0  BranchType=C  Resistance=RReiheL3  Inductance=2.4e-3  SetiL0=off  InitialCurrent=0  Capacitance=C_Zwischenkreis  Setx0=off  InitialVoltage=700  Measurements=None
  I A: : powerlib/Measurements/Current Measurement  PhasorSimulation=off  OutputType=Complex  PSBequivalent=0
  I A:1 : powerlib/Measurements/Current Measurement  PhasorSimulation=off  OutputType=Complex  PSBequivalent=0
  Series RLC Branch2 : powerlib/Elements/Series RLC Branch  LConnTagsString=__new0  RConnTagsString=__new0  BranchType=R  Resistance=40e3  Inductance=2.4e-3  SetiL0=off  InitialCurrent=0  Capacitance=C_Zwischenkreis  Setx0=off  InitialVoltage=0  Measurements=None
  U DC: : powerlib/Measurements/Voltage Measurement  PhasorSimulation=off  OutputType=Complex  PSBequivalent=0
  DC+ out : PMIOPort  Side=Right
  DC- out : PMIOPort  Port=2  Side=Right
  DC+ in : PMIOPort  Port=3  Side=Left
  DC- in : PMIOPort  Port=4  Side=Left
  U DC Zwischenkreis : Outport
  I DC Zwischenkreis in : Outport  Port=2
  I DC Zwischenkreis out : Outport  Port=3
  wires:
  U DC:/1 -> U DC Zwischenkreis/1
  I A:/1 -> I DC Zwischenkreis in/1
  I A:1/1 -> I DC Zwischenkreis out/1
  connections:
  C Zwischenkreis/LConn1 -- I A:/RConn1 -- I A:1/LConn1 -- U DC:/LConn1 -- Series RLC Branch2/LConn1
  DC- out/RConn1 -- U DC:/LConn2 -- DC- in/RConn1 -- C Zwischenkreis/RConn1 -- Series RLC Branch2/RConn1
  DC+ in/RConn1 -- I A:/LConn1
  DC+ out/RConn1 -- I A:1/RConn1
